simulink model "state_feedback_discrete"  (R2015b)
settings: Solver=VariableStepAuto  StartTime=0.0  StopTime=t  RelTol=1e-3
values from neighbouring files (symbols this model uses):
  A12 = A(1:3,4:6)    [StateSpace.m]
  F = Fe(:,1:size(A,2))    [StateSpace.m]
  FI = Fe(:,size(A,2)+1:size(Fe,2))    [StateSpace.m]
  Jx = 0.0107    [Parameters.m]
  Jy = 0.0107    [Parameters.m]
  Jz = 0.02135    [Parameters.m]
  kd = 9.39741e-7    (= 9.39741e-07)    [Parameters.m]
  kth = 1.32922e-5    (= 1.32922e-05)    [Parameters.m]
  L = 0.225    [Parameters.m]
  Lobs = (-place(A22',A12',[-20 -25 -30]))'    [StateSpace.m]
  pitch_ref = 0.5    [plotSim.m]
  pitch_time = 2    [plotSim.m]
  roll_ref = 0.5    [plotSim.m]
  roll_time = 0.5    [plotSim.m]
  T = 0.035    [plotSim.m]
  w2_bar = sqrt(Fg/kth/4)+1    [Parameters.m]
  w3_bar = sqrt(Fg/kth/4)+1    [Parameters.m]
  w4_bar = sqrt(Fg/kth/4)+1    [Parameters.m]
  yaw_ref = 0.5    [plotSim.m]
  yaw_time = 4    [plotSim.m]
settings Model: Creator=USUARIO  LastModifiedBy=USUARIO

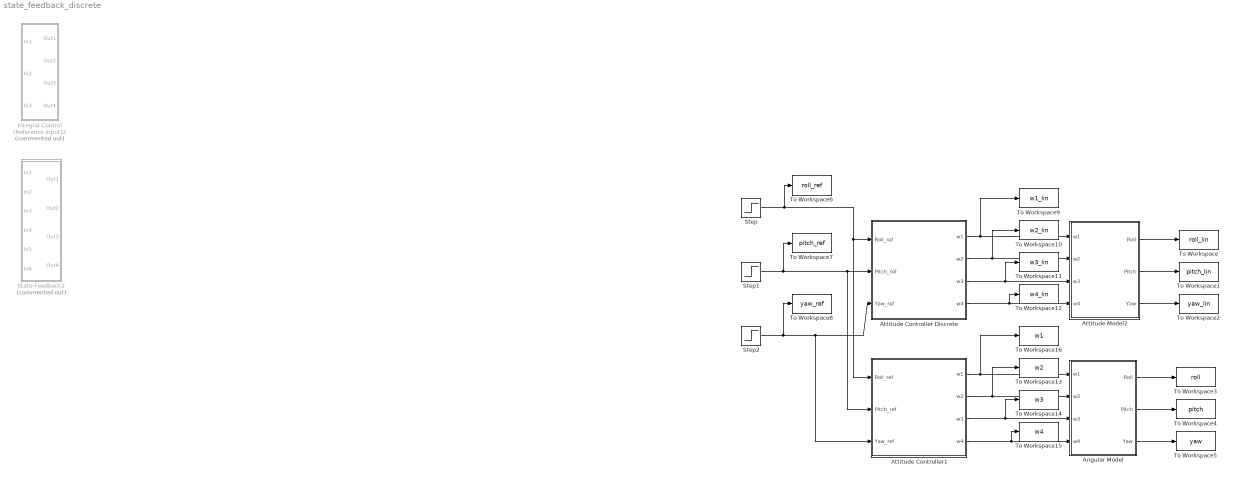
== system state_feedback_discrete ==
  Angular Model : Subsystem
  Attitude Controller Discrete : Subsystem
  Attitude Controller1 : Subsystem
  "Attitude Model2 " : Subsystem
  Integral Control (Reference Input)2 : Subsystem  Commented=on
  State-Feedback2 : Subsystem  Commented=on
  Step : Step  Time=roll_time  After=roll_ref  SampleTime=0
  Step1 : Step  Time=pitch_time  After=pitch_ref  SampleTime=0
  Step2 : Step  Time=yaw_time  After=yaw_ref  SampleTime=0
  To Workspace : ToWorkspace  VariableName=roll_lin  SaveFormat=Timeseries  SampleTime=-1
  To Workspace1 : ToWorkspace  VariableName=pitch_lin  SaveFormat=Timeseries  SampleTime=-1
  To Workspace10 : ToWorkspace  VariableName=w2_lin  SaveFormat=Timeseries  SampleTime=-1
  To Workspace11 : ToWorkspace  VariableName=w3_lin  SaveFormat=Timeseries  SampleTime=-1
  To Workspace12 : ToWorkspace  VariableName=w4_lin  SaveFormat=Timeseries  SampleTime=-1
  To Workspace13 : ToWorkspace  VariableName=w2  SaveFormat=Timeseries  SampleTime=-1
  To Workspace14 : ToWorkspace  VariableName=w3  SaveFormat=Timeseries  SampleTime=-1
  To Workspace15 : ToWorkspace  VariableName=w4  SaveFormat=Timeseries  SampleTime=-1
  To Workspace16 : ToWorkspace  VariableName=w1  SaveFormat=Timeseries  SampleTime=-1
  To Workspace2 : ToWorkspace  VariableName=yaw_lin  SaveFormat=Timeseries  SampleTime=-1
  To Workspace3 : ToWorkspace  VariableName=roll  SaveFormat=Timeseries  SampleTime=-1
  To Workspace4 : ToWorkspace  VariableName=pitch  SaveFormat=Timeseries  SampleTime=-1
  To Workspace5 : ToWorkspace  VariableName=yaw  SaveFormat=Timeseries  SampleTime=-1
  To Workspace6 : ToWorkspace  VariableName=roll_ref  SaveFormat=Timeseries  SampleTime=-1
  To Workspace7 : ToWorkspace  VariableName=pitch_ref  SaveFormat=Timeseries  SampleTime=-1
  To Workspace8 : ToWorkspace  VariableName=yaw_ref  SaveFormat=Timeseries  SampleTime=-1
  To Workspace9 : ToWorkspace  VariableName=w1_lin  SaveFormat=Timeseries  SampleTime=-1
  wires:
  Attitude Controller Discrete/3(w3) -> "Attitude Model2 "/3(w3), To Workspace11/1
  Attitude Controller Discrete/2(w2) -> To Workspace10/1, "Attitude Model2 "/2(w2)
  Attitude Controller Discrete/1(w1) -> To Workspace9/1, "Attitude Model2 "/1(w1)
  Attitude Controller Discrete/4(w4) -> "Attitude Model2 "/4(w4), To Workspace12/1
  "Attitude Model2 "/2(Pitch) -> To Workspace1/1
  "Attitude Model2 "/1(Roll) -> To Workspace/1
  "Attitude Model2 "/3(Yaw) -> To Workspace2/1
  Step/1 -> Attitude Controller1/1(Roll_ref), Attitude Controller Discrete/1(Roll_ref), To Workspace6/1
  Step1/1 -> Attitude Controller1/2(Pitch_ref), Attitude Controller Discrete/2(Pitch_ref), To Workspace7/1
  Step2/1 -> Attitude Controller1/3(Yaw_ref), Attitude Controller Discrete/3(Yaw_ref), To Workspace8/1
  Angular Model/3(Yaw) -> To Workspace5/1
  Angular Model/2(Pitch) -> To Workspace4/1
  Angular Model/1(Roll) -> To Workspace3/1
  Attitude Controller1/3(w3) -> Angular Model/3(w3), To Workspace14/1
  Attitude Controller1/2(w2) -> Angular Model/2(w2), To Workspace13/1
  Attitude Controller1/1(w1) -> To Workspace16/1, Angular Model/1(w1)
  Attitude Controller1/4(w4) -> To Workspace15/1, Angular Model/4(w4)

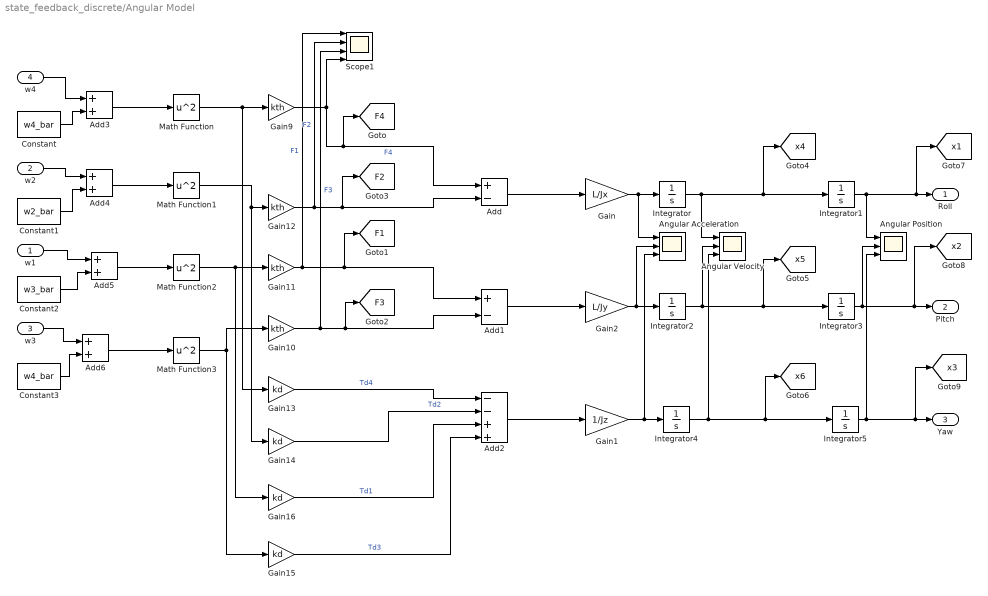
== system state_feedback_discrete/Angular Model ==
  w1 : Inport
  w2 : Inport  Port=2
  w3 : Inport  Port=3
  w4 : Inport  Port=4
  Add : Sum  Inputs=+-
  Add1 : Sum  Inputs=+-
  Add2 : Sum  Inputs=--++
  Add{3..6} (4 alike) : Sum
  Angular Position : Scope  NumInputPorts=3
  Angular Velocity : Scope  NumInputPorts=3
  Angular Acceleration : Scope  NumInputPorts=3
  Constant : Constant  Value=w4_bar
  Constant1 : Constant  Value=w2_bar
  Constant2 : Constant  Value=w3_bar
  Constant3 : Constant  Value=w4_bar
  Gain : Gain  Gain=L/Jx
  Gain1 : Gain  Gain=1/Jz
  Gain{9..12} (4 alike) : Gain  Gain=kth
  Gain{13..16} (4 alike) : Gain  Gain=kd
  Gain2 : Gain  Gain=L/Jy
  Integrator{,1..5} (6 alike) : Integrator
  Math Function{,1..3} (4 alike) : Math  Operator=square  SaturateOnIntegerOverflow=on
  Scope1 : Scope  NumInputPorts=4
  Roll : Outport
  Pitch : Outport  Port=2
  Yaw : Outport  Port=3
  tag scope: F1=global, F2=global, F3=global, F4=global, x1=global, x2=global, x3=global, x4=global, x5=global, x6=global
  wires:
  Gain2/1 -> Angular Acceleration/2, Integrator2/1
  Add2/1 -> Gain1/1
  Gain9/1 -> [F4], Add/1, Scope1/4  "F4"
  Gain14/1 -> Add2/2  "Td2"
  Gain16/1 -> Add2/3  "Td1"
  Gain/1 -> Angular Acceleration/1, Integrator/1
  Integrator/1 -> Angular Velocity/1, Integrator1/1, [x4]
  Integrator1/1 -> [x1], Roll/1, Angular Position/1
  Integrator4/1 -> Angular Velocity/3, [x6], Integrator5/1
  Add/1 -> Gain/1
  Integrator3/1 -> [x2], Pitch/1, Angular Position/2
  Add1/1 -> Gain2/1
  Integrator5/1 -> Angular Position/3, [x3], Yaw/1
  Gain12/1 -> Scope1/2, [F2], Add/2  "F2"
  Gain10/1 -> [F3], Add1/2, Scope1/3  "F3"
  Gain11/1 -> Scope1/1, [F1], Add1/1  "F1"
  Gain13/1 -> Add2/1  "Td4"
  Gain15/1 -> Add2/4  "Td3"
  Integrator2/1 -> Angular Velocity/2, [x5], Integrator3/1
  Gain1/1 -> Angular Acceleration/3, Integrator4/1
  Math Function3/1 -> Gain10/1, Gain15/1
  Math Function2/1 -> Gain16/1, Gain11/1
  Math Function/1 -> Gain13/1, Gain9/1
  Math Function1/1 -> Gain14/1, Gain12/1
  w4/1 -> Add3/1
  Add3/1 -> Math Function/1
  Constant/1 -> Add3/2
  w2/1 -> Add4/1
  Add4/1 -> Math Function1/1
  Constant1/1 -> Add4/2
  w1/1 -> Add5/1
  Add5/1 -> Math Function2/1
  Constant2/1 -> Add5/2
  w3/1 -> Add6/1
  Add6/1 -> Math Function3/1
  Constant3/1 -> Add6/2

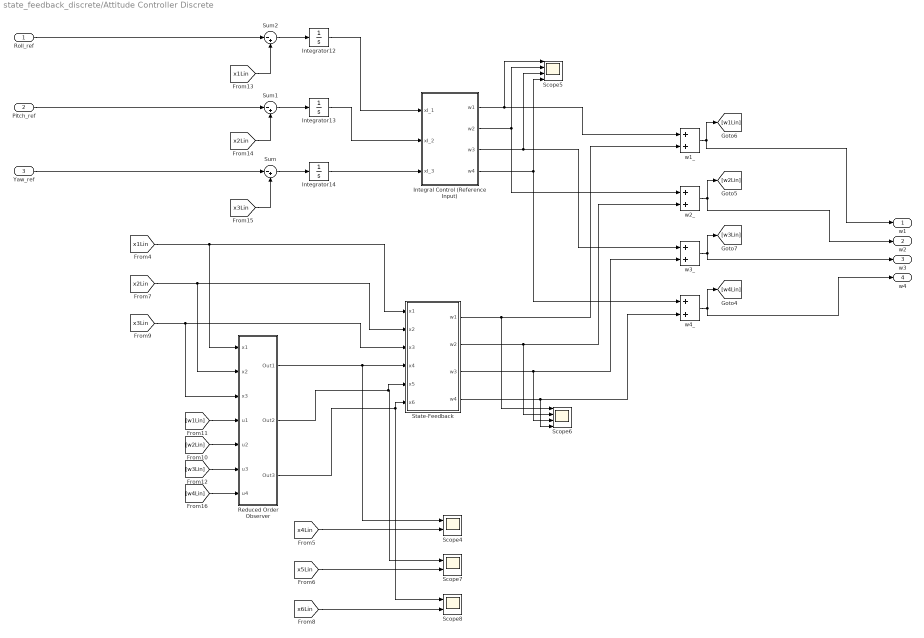
== system state_feedback_discrete/Attitude Controller Discrete ==
  Roll_ref : Inport
  Pitch_ref : Inport  Port=2
  Yaw_ref : Inport  Port=3
  Integral Control (Reference Input) : MATLAB Function  TreatAsAtomicUnit=on
  Integrator12 : Integrator
  Integrator13 : Integrator
  Integrator14 : Integrator
  Reduced Order Observer : Subsystem
  Scope4 : Scope  NumInputPorts=2
  Scope5 : Scope  NumInputPorts=4
  Scope6 : Scope  NumInputPorts=4
  Scope7 : Scope  NumInputPorts=2
  Scope8 : Scope  NumInputPorts=2
  "State-Feedback " : MATLAB Function  TreatAsAtomicUnit=on
  Sum : Sum  Inputs=|-+
  Sum1 : Sum  Inputs=|-+
  Sum2 : Sum  Inputs=|-+
  w1_ : Sum
  w2_ : Sum
  w3_ : Sum
  w4_ : Sum
  w1 : Outport
  w2 : Outport  Port=2
  w3 : Outport  Port=3
  w4 : Outport  Port=4
  wires:
  "State-Feedback "/4(w4) -> w4_/2, Scope6/4
  Roll_ref/1 -> Sum2/1
  [x3Lin] -> Sum/2
  [x1Lin] -> Sum2/2
  Integrator13/1 -> Integral Control (Reference Input)/2(xI_2)
  "State-Feedback "/1(w1) -> w1_/2, Scope6/1
  [w3Lin] -> Reduced Order Observer/6(u3)
  Sum2/1 -> Integrator12/1
  Sum/1 -> Integrator14/1
  [x3Lin] -> "State-Feedback "/3(x3), Reduced Order Observer/3(x3)
  [w2Lin] -> Reduced Order Observer/5(u2)
  Pitch_ref/1 -> Sum1/1
  Integrator14/1 -> Integral Control (Reference Input)/3(xI_3)
  Reduced Order Observer/3(Out3) -> "State-Feedback "/6(x6), Scope8/1
  [x4Lin] -> Scope4/2
  [x6Lin] -> Scope8/2
  "State-Feedback "/2(w2) -> w2_/2, Scope6/2
  Integral Control (Reference Input)/2(w2) -> Scope5/2, w2_/1
  [w4Lin] -> Reduced Order Observer/7(u4)
  Integral Control (Reference Input)/3(w3) -> w3_/1, Scope5/3
  Reduced Order Observer/2(Out2) -> "State-Feedback "/5(x5), Scope7/1
  [x1Lin] -> "State-Feedback "/1(x1), Reduced Order Observer/1(x1)
  [w1Lin] -> Reduced Order Observer/4(u1)
  Integrator12/1 -> Integral Control (Reference Input)/1(xI_1)
  [x2Lin] -> Sum1/2
  Integral Control (Reference Input)/4(w4) -> Scope5/4, w4_/1
  Integral Control (Reference Input)/1(w1) -> w1_/1, Scope5/1
  [x2Lin] -> "State-Feedback "/2(x2), Reduced Order Observer/2(x2)
  Reduced Order Observer/1(Out1) -> "State-Feedback "/4(x4), Scope4/1
  [x5Lin] -> Scope7/2
  Sum1/1 -> Integrator13/1
  Yaw_ref/1 -> Sum/1
  "State-Feedback "/3(w3) -> w3_/2, Scope6/3
  w1_/1 -> w1/1, [w1Lin]
  w4_/1 -> w4/1, [w4Lin]
  w2_/1 -> w2/1, [w2Lin]
  w3_/1 -> w3/1, [w3Lin]

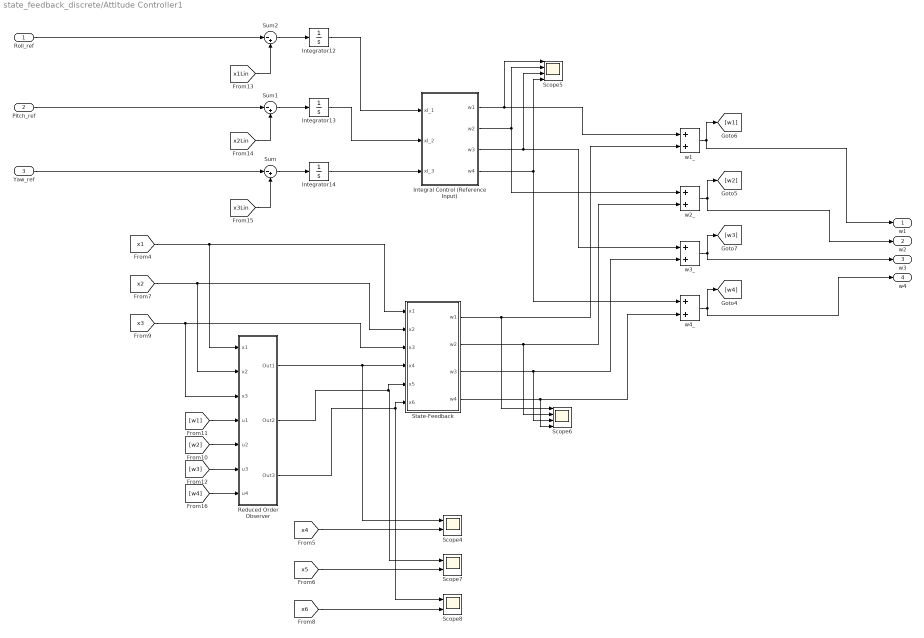
== system state_feedback_discrete/Attitude Controller1 ==
  Roll_ref : Inport
  Pitch_ref : Inport  Port=2
  Yaw_ref : Inport  Port=3
  Integral Control (Reference Input) : MATLAB Function  TreatAsAtomicUnit=on
  Integrator12 : Integrator
  Integrator13 : Integrator
  Integrator14 : Integrator
  Reduced Order Observer : Subsystem
  Scope4 : Scope  NumInputPorts=2
  Scope5 : Scope  NumInputPorts=4
  Scope6 : Scope  NumInputPorts=4
  Scope7 : Scope  NumInputPorts=2
  Scope8 : Scope  NumInputPorts=2
  "State-Feedback " : MATLAB Function  TreatAsAtomicUnit=on
  Sum : Sum  Inputs=|-+
  Sum1 : Sum  Inputs=|-+
  Sum2 : Sum  Inputs=|-+
  w1_ : Sum
  w2_ : Sum
  w3_ : Sum
  w4_ : Sum
  w1 : Outport
  w2 : Outport  Port=2
  w3 : Outport  Port=3
  w4 : Outport  Port=4
  wires:
  w3_/1 -> [w3], w3/1
  w2_/1 -> [w2], w2/1
  w4_/1 -> [w4], w4/1
  w1_/1 -> [w1], w1/1
  "State-Feedback "/3(w3) -> Scope6/3, w3_/2
  Yaw_ref/1 -> Sum/1
  Sum1/1 -> Integrator13/1
  [x5] -> Scope7/2
  Reduced Order Observer/1(Out1) -> Scope4/1, "State-Feedback "/4(x4)
  [x2] -> Reduced Order Observer/2(x2), "State-Feedback "/2(x2)
  Integral Control (Reference Input)/1(w1) -> Scope5/1, w1_/1
  Integral Control (Reference Input)/4(w4) -> w4_/1, Scope5/4
  [x2Lin] -> Sum1/2
  Integrator12/1 -> Integral Control (Reference Input)/1(xI_1)
  [w1] -> Reduced Order Observer/4(u1)
  [x1] -> Reduced Order Observer/1(x1), "State-Feedback "/1(x1)
  Reduced Order Observer/2(Out2) -> Scope7/1, "State-Feedback "/5(x5)
  Integral Control (Reference Input)/3(w3) -> Scope5/3, w3_/1
  [w4] -> Reduced Order Observer/7(u4)
  Integral Control (Reference Input)/2(w2) -> w2_/1, Scope5/2
  "State-Feedback "/2(w2) -> Scope6/2, w2_/2
  [x6] -> Scope8/2
  [x4] -> Scope4/2
  Reduced Order Observer/3(Out3) -> Scope8/1, "State-Feedback "/6(x6)
  Integrator14/1 -> Integral Control (Reference Input)/3(xI_3)
  Pitch_ref/1 -> Sum1/1
  [w2] -> Reduced Order Observer/5(u2)
  [x3] -> Reduced Order Observer/3(x3), "State-Feedback "/3(x3)
  Sum/1 -> Integrator14/1
  Sum2/1 -> Integrator12/1
  [w3] -> Reduced Order Observer/6(u3)
  "State-Feedback "/1(w1) -> Scope6/1, w1_/2
  Integrator13/1 -> Integral Control (Reference Input)/2(xI_2)
  [x1Lin] -> Sum2/2
  [x3Lin] -> Sum/2
  Roll_ref/1 -> Sum2/1
  "State-Feedback "/4(w4) -> Scope6/4, w4_/2

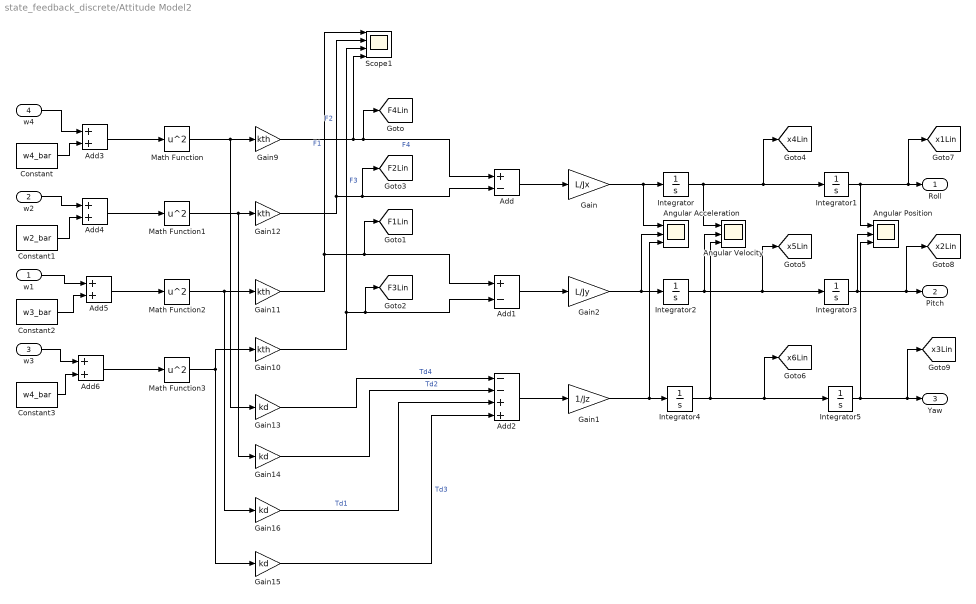
== system state_feedback_discrete/Attitude Model2  ==
  w1 : Inport
  w2 : Inport  Port=2
  w3 : Inport  Port=3
  w4 : Inport  Port=4
  Add : Sum  Inputs=+-
  Add1 : Sum  Inputs=+-
  Add2 : Sum  Inputs=--++
  Add{3..6} (4 alike) : Sum
  Angular Position : Scope  NumInputPorts=3
  Angular Velocity : Scope  NumInputPorts=3
  Angular Acceleration : Scope  NumInputPorts=3
  Constant : Constant  Value=w4_bar
  Constant1 : Constant  Value=w2_bar
  Constant2 : Constant  Value=w3_bar
  Constant3 : Constant  Value=w4_bar
  Gain : Gain  Gain=L/Jx
  Gain1 : Gain  Gain=1/Jz
  Gain{9..12} (4 alike) : Gain  Gain=kth
  Gain{13..16} (4 alike) : Gain  Gain=kd
  Gain2 : Gain  Gain=L/Jy
  Integrator{,1..5} (6 alike) : Integrator
  Math Function{,1..3} (4 alike) : Math  Operator=square  SaturateOnIntegerOverflow=on
  Scope1 : Scope  NumInputPorts=4
  Roll : Outport
  Pitch : Outport  Port=2
  Yaw : Outport  Port=3
  tag scope: F1Lin=global, F2Lin=global, F3Lin=global, F4Lin=global, x1Lin=global, x2Lin=global, x3Lin=global, x4Lin=global, x5Lin=global, x6Lin=global
  wires:
  Gain1/1 -> Integrator4/1, Angular Acceleration/3
  Integrator2/1 -> Integrator3/1, [x5Lin], Angular Velocity/2
  Gain15/1 -> Add2/4  "Td3"
  Gain13/1 -> Add2/1  "Td4"
  Gain11/1 -> Add1/1, [F1Lin], Scope1/1  "F1"
  Gain10/1 -> Scope1/3, Add1/2, [F3Lin]  "F3"
  Gain12/1 -> Scope1/2, Add/2, [F2Lin]  "F2"
  Integrator5/1 -> Yaw/1, [x3Lin], Angular Position/3
  Add1/1 -> Gain2/1
  Integrator3/1 -> Angular Position/2, Pitch/1, [x2Lin]
  Add/1 -> Gain/1
  Integrator4/1 -> Integrator5/1, [x6Lin], Angular Velocity/3
  Integrator1/1 -> Angular Position/1, Roll/1, [x1Lin]
  Integrator/1 -> [x4Lin], Integrator1/1, Angular Velocity/1
  Gain/1 -> Integrator/1, Angular Acceleration/1
  Gain16/1 -> Add2/3  "Td1"
  Gain14/1 -> Add2/2  "Td2"
  Gain9/1 -> Scope1/4, Add/1, [F4Lin]  "F4"
  Add2/1 -> Gain1/1
  Gain2/1 -> Integrator2/1, Angular Acceleration/2
  Math Function3/1 -> Gain10/1, Gain15/1
  Math Function2/1 -> Gain16/1, Gain11/1
  Math Function/1 -> Gain13/1, Gain9/1
  Math Function1/1 -> Gain14/1, Gain12/1
  w4/1 -> Add3/1
  Add3/1 -> Math Function/1
  Constant/1 -> Add3/2
  w2/1 -> Add4/1
  Add4/1 -> Math Function1/1
  Constant1/1 -> Add4/2
  w1/1 -> Add5/1
  Add5/1 -> Math Function2/1
  Constant2/1 -> Add5/2
  w3/1 -> Add6/1
  Add6/1 -> Math Function3/1
  Constant3/1 -> Add6/2

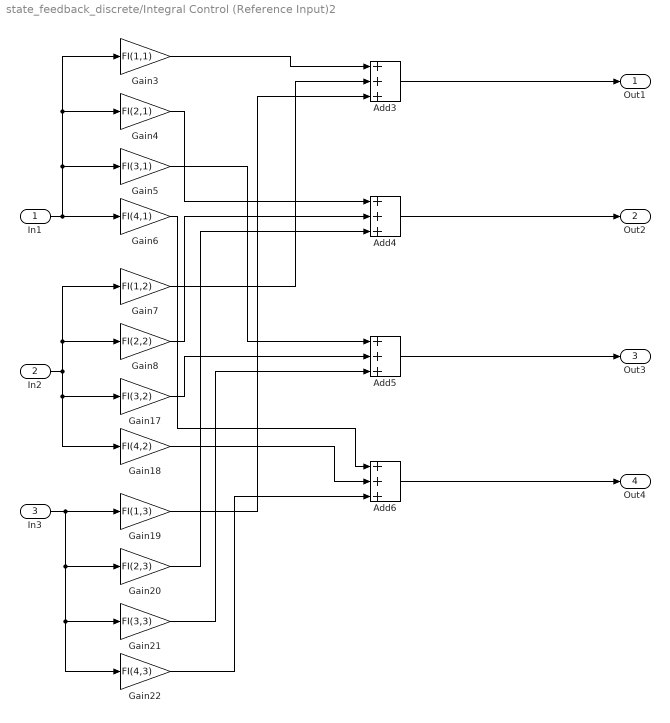
== system state_feedback_discrete/Integral Control (Reference Input)2 ==
  In1 : Inport
  In2 : Inport  Port=2
  In3 : Inport  Port=3
  Add{3..6} (4 alike) : Sum  Inputs=+++
  Gain17 : Gain  Gain=FI(3,2)
  Gain18 : Gain  Gain=FI(4,2)
  Gain19 : Gain  Gain=FI(1,3)
  Gain20 : Gain  Gain=FI(2,3)
  Gain21 : Gain  Gain=FI(3,3)
  Gain22 : Gain  Gain=FI(4,3)
  Gain3 : Gain  Gain=FI(1,1)
  Gain4 : Gain  Gain=FI(2,1)
  Gain5 : Gain  Gain=FI(3,1)
  Gain6 : Gain  Gain=FI(4,1)
  Gain7 : Gain  Gain=FI(1,2)
  Gain8 : Gain  Gain=FI(2,2)
  Out1 : Outport
  Out2 : Outport  Port=2
  Out3 : Outport  Port=3
  Out4 : Outport  Port=4
  wires:
  Gain21/1 -> Add5/3
  Gain17/1 -> Add5/2
  Gain5/1 -> Add5/1
  Gain6/1 -> Add6/1
  Gain22/1 -> Add6/3
  Gain18/1 -> Add6/2
  In2/1 -> Gain7/1, Gain8/1, Gain17/1, Gain18/1
  Add5/1 -> Out3/1
  Add6/1 -> Out4/1
  In3/1 -> Gain19/1, Gain20/1, Gain22/1, Gain21/1
  Add3/1 -> Out1/1
  Add4/1 -> Out2/1
  Gain20/1 -> Add4/3
  Gain3/1 -> Add3/1
  Gain19/1 -> Add3/3
  Gain7/1 -> Add3/2
  Gain8/1 -> Add4/2
  Gain4/1 -> Add4/1
  In1/1 -> Gain3/1, Gain4/1, Gain5/1, Gain6/1

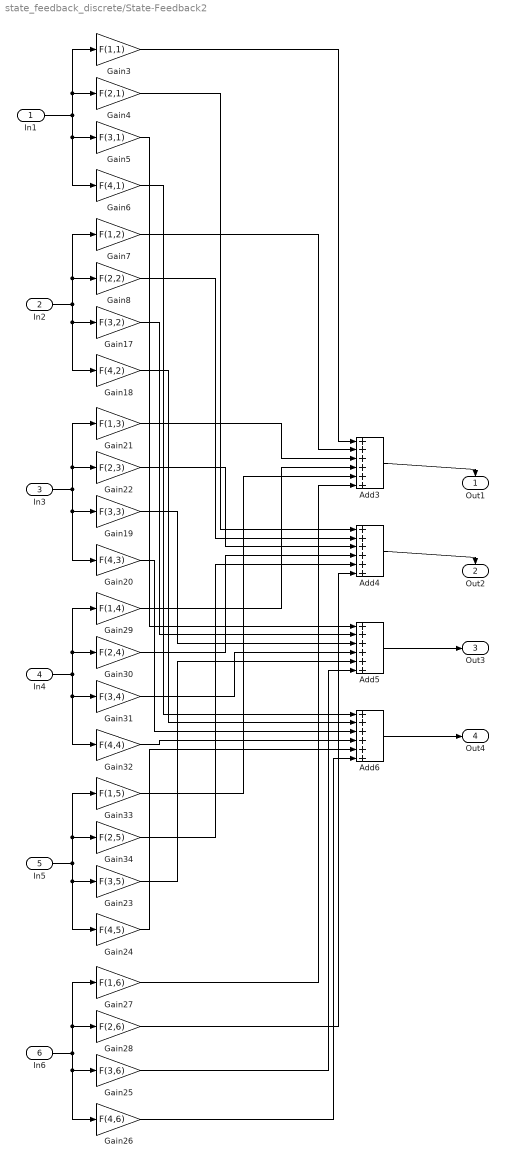
== system state_feedback_discrete/State-Feedback2 ==
  In1 : Inport
  In2 : Inport  Port=2
  In3 : Inport  Port=3
  In4 : Inport  Port=4
  In5 : Inport  Port=5
  In6 : Inport  Port=6
  Add{3..6} (4 alike) : Sum  Inputs=++++++
  Gain17 : Gain  Gain=F(3,2)
  Gain18 : Gain  Gain=F(4,2)
  Gain19 : Gain  Gain=F(3,3)
  Gain20 : Gain  Gain=F(4,3)
  Gain21 : Gain  Gain=F(1,3)
  Gain22 : Gain  Gain=F(2,3)
  Gain23 : Gain  Gain=F(3,5)
  Gain24 : Gain  Gain=F(4,5)
  Gain25 : Gain  Gain=F(3,6)
  Gain26 : Gain  Gain=F(4,6)
  Gain27 : Gain  Gain=F(1,6)
  Gain28 : Gain  Gain=F(2,6)
  Gain29 : Gain  Gain=F(1,4)
  Gain3 : Gain  Gain=F(1,1)
  Gain30 : Gain  Gain=F(2,4)
  Gain31 : Gain  Gain=F(3,4)
  Gain32 : Gain  Gain=F(4,4)
  Gain33 : Gain  Gain=F(1,5)
  Gain34 : Gain  Gain=F(2,5)
  Gain4 : Gain  Gain=F(2,1)
  Gain5 : Gain  Gain=F(3,1)
  Gain6 : Gain  Gain=F(4,1)
  Gain7 : Gain  Gain=F(1,2)
  Gain8 : Gain  Gain=F(2,2)
  Out1 : Outport
  Out2 : Outport  Port=2
  Out3 : Outport  Port=3
  Out4 : Outport  Port=4
  wires:
  In2/1 -> Gain8/1, Gain7/1, Gain18/1, Gain17/1
  In1/1 -> Gain6/1, Gain5/1, Gain4/1, Gain3/1
  In3/1 -> Gain22/1, Gain21/1, Gain20/1, Gain19/1
  In5/1 -> Gain34/1, Gain33/1, Gain24/1, Gain23/1
  In4/1 -> Gain32/1, Gain31/1, Gain30/1, Gain29/1
  In6/1 -> Gain28/1, Gain27/1, Gain26/1, Gain25/1
  Add3/1 -> Out1/1
  Add4/1 -> Out2/1
  Add5/1 -> Out3/1
  Add6/1 -> Out4/1
  Gain4/1 -> Add4/1
  Gain22/1 -> Add4/3
  Gain8/1 -> Add4/2
  Gain34/1 -> Add4/5
  Gain30/1 -> Add4/4
  Gain28/1 -> Add4/6
  Gain24/1 -> Add6/5
  Gain20/1 -> Add6/3
  Gain6/1 -> Add6/1
  Gain18/1 -> Add6/2
  Gain26/1 -> Add6/6
  Gain32/1 -> Add6/4
  Gain7/1 -> Add3/2
  Gain21/1 -> Add3/3
  Gain29/1 -> Add3/4
  Gain27/1 -> Add3/6
  Gain3/1 -> Add3/1
  Gain33/1 -> Add3/5
  Gain23/1 -> Add5/5
  Gain17/1 -> Add5/2
  Gain19/1 -> Add5/3
  Gain5/1 -> Add5/1
  Gain31/1 -> Add5/4
  Gain25/1 -> Add5/6

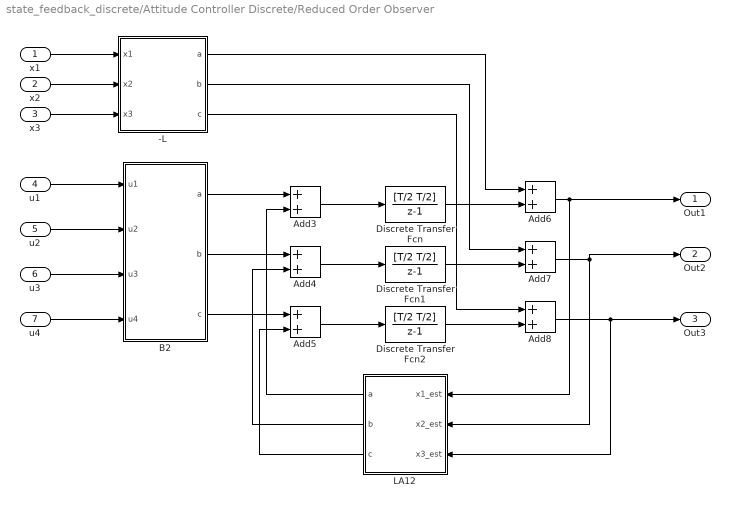
== system state_feedback_discrete/Attitude Controller Discrete/Reduced Order Observer ==
  x1 : Inport
  x2 : Inport  Port=2
  x3 : Inport  Port=3
  u1 : Inport  Port=4
  u2 : Inport  Port=5
  u3 : Inport  Port=6
  u4 : Inport  Port=7
  "-L " : MATLAB Function  TreatAsAtomicUnit=on
  Add{3..8} (6 alike) : Sum  Inputs=2
  B2 : MATLAB Function  TreatAsAtomicUnit=on
  Discrete Transfer Fcn : DiscreteTransferFcn  Numerator=[T/2 T/2]  Denominator=[1 -1]  SampleTime=T
  Discrete Transfer Fcn1 : DiscreteTransferFcn  Numerator=[T/2 T/2]  Denominator=[1 -1]  SampleTime=T
  Discrete Transfer Fcn2 : DiscreteTransferFcn  Numerator=[T/2 T/2]  Denominator=[1 -1]  SampleTime=T
  LA12 : MATLAB Function  TreatAsAtomicUnit=on
  Out1 : Outport
  Out2 : Outport  Port=2
  Out3 : Outport  Port=3
  wires:
  Add4/1 -> Discrete Transfer Fcn1/1
  Add3/1 -> Discrete Transfer Fcn/1
  Add5/1 -> Discrete Transfer Fcn2/1
  u4/1 -> B2/4(u4)
  u2/1 -> B2/2(u2)
  B2/1(a) -> Add3/1
  B2/2(b) -> Add4/1
  B2/3(c) -> Add5/1
  LA12/1(a) -> Add3/2
  LA12/2(b) -> Add4/2
  LA12/3(c) -> Add5/2
  Add6/1 -> LA12/1(x1_est), Out1/1
  Add7/1 -> LA12/2(x2_est), Out2/1
  Add8/1 -> LA12/3(x3_est), Out3/1
  "-L "/3(c) -> Add8/1
  "-L "/1(a) -> Add6/1
  "-L "/2(b) -> Add7/1
  x2/1 -> "-L "/2(x2)
  x3/1 -> "-L "/3(x3)
  x1/1 -> "-L "/1(x1)
  u1/1 -> B2/1(u1)
  u3/1 -> B2/3(u3)
  Discrete Transfer Fcn/1 -> Add6/2
  Discrete Transfer Fcn1/1 -> Add7/2
  Discrete Transfer Fcn2/1 -> Add8/2

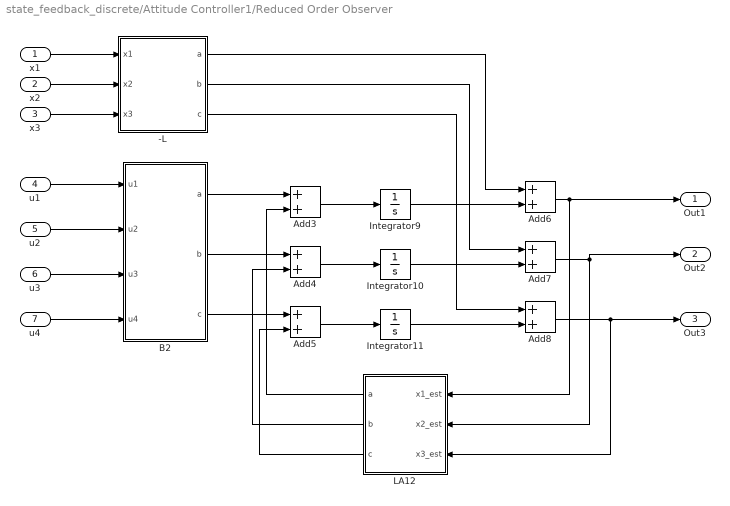
== system state_feedback_discrete/Attitude Controller1/Reduced Order Observer ==
  x1 : Inport
  x2 : Inport  Port=2
  x3 : Inport  Port=3
  u1 : Inport  Port=4
  u2 : Inport  Port=5
  u3 : Inport  Port=6
  u4 : Inport  Port=7
  "-L " : MATLAB Function  TreatAsAtomicUnit=on
  Add{3..8} (6 alike) : Sum  Inputs=2
  B2 : MATLAB Function  TreatAsAtomicUnit=on
  Integrator10 : Integrator
  Integrator11 : Integrator
  Integrator9 : Integrator
  LA12 : MATLAB Function  TreatAsAtomicUnit=on
  Out1 : Outport
  Out2 : Outport  Port=2
  Out3 : Outport  Port=3
  wires:
  u3/1 -> B2/3(u3)
  u1/1 -> B2/1(u1)
  Integrator10/1 -> Add7/2
  Integrator11/1 -> Add8/2
  Integrator9/1 -> Add6/2
  x1/1 -> "-L "/1(x1)
  x3/1 -> "-L "/3(x3)
  x2/1 -> "-L "/2(x2)
  "-L "/2(b) -> Add7/1
  "-L "/1(a) -> Add6/1
  "-L "/3(c) -> Add8/1
  Add8/1 -> Out3/1, LA12/3(x3_est)
  Add7/1 -> Out2/1, LA12/2(x2_est)
  Add6/1 -> Out1/1, LA12/1(x1_est)
  LA12/3(c) -> Add5/2
  LA12/2(b) -> Add4/2
  LA12/1(a) -> Add3/2
  B2/3(c) -> Add5/1
  B2/2(b) -> Add4/1
  B2/1(a) -> Add3/1
  u2/1 -> B2/2(u2)
  u4/1 -> B2/4(u4)
  Add5/1 -> Integrator11/1
  Add3/1 -> Integrator9/1
  Add4/1 -> Integrator10/1

== matlab function state_feedback_discrete/Attitude Controller1/Integral Control (Reference Input) ==
  data: xI_1 input; w1 output; w2 output; w3 output; w4 output; xI_2 input; xI_3 input; FI parameter
function [w1,w2,w3,w4] = FI_matrix(xI_1, xI_2, xI_3,FI)
xI=[xI_1;
    xI_2;
    xI_3];

w=FI*xI;

w1=w(1);
w2=w(2);
w3=w(3);
w4=w(4);

== matlab function state_feedback_discrete/Attitude Controller1/Reduced Order Observer/-L  ==
  data: x1 input; a output; b output; c output; x2 input; x3 input; Lobs parameter
function [a,b,c] = minusL_matrix(x1, x2, x3, Lobs)
x=[x1;
    x2;
    x3];

abc=-Lobs*x;

a=abc(1);
b=abc(2);
c=abc(3);

== matlab function state_feedback_discrete/Attitude Controller1/Reduced Order Observer/B2 ==
  data: u1 input; a output; b output; c output; u2 input; u3 input; u4 input; B2 parameter
function [a, b, c] = B2_matrix(u1, u2, u3, u4, B2)
u=[u1;
    u2;
    u3;
    u4];

abc=B2*u;

a=abc(1);
b=abc(2);
c=abc(3);

== matlab function state_feedback_discrete/Attitude Controller1/Reduced Order Observer/LA12 ==
  data: x1_est input; x2_est input; x3_est input; a output; b output; c output; Lobs parameter; A12 parameter
function [a,b,c] = LA12_matrix(x1_est, x2_est, x3_est, Lobs, A12)
x=[x1_est;
    x2_est;
    x3_est];

abc=Lobs*A12*x;

a=abc(1);
b=abc(2);
c=abc(3);

== matlab function state_feedback_discrete/Attitude Controller1/State-Feedback  ==
  data: x1 input; w1 output; w2 output; w3 output; w4 output; x2 input; x3 input; x4 input; x5 input; x6 input; F parameter
function [w1,w2,w3,w4] = F_matrix(x1, x2, x3, x4, x5, x6, F)
x=[x1;
    x2;
    x3;
    x4;
    x5;
    x6];

w=F*x;

w1=w(1);
w2=w(2);
w3=w(3);
w4=w(4);

== matlab function state_feedback_discrete/Attitude Controller Discrete/Integral Control (Reference Input) ==
  data: xI_1 input; w1 output; w2 output; w3 output; w4 output; xI_2 input; xI_3 input; FI parameter
function [w1,w2,w3,w4] = FI_matrix(xI_1, xI_2, xI_3,FI)
xI=[xI_1;
    xI_2;
    xI_3];

w=FI*xI;

w1=w(1);
w2=w(2);
w3=w(3);
w4=w(4);

== matlab function state_feedback_discrete/Attitude Controller Discrete/Reduced Order Observer/-L  ==
  data: x1 input; a output; b output; c output; x2 input; x3 input; Lobs parameter
function [a,b,c] = minusL_matrix(x1, x2, x3, Lobs)
x=[x1;
    x2;
    x3];

abc=-Lobs*x;

a=abc(1);
b=abc(2);
c=abc(3);

== matlab function state_feedback_discrete/Attitude Controller Discrete/Reduced Order Observer/B2 ==
  data: u1 input; a output; b output; c output; u2 input; u3 input; u4 input; B2 parameter
function [a, b, c] = B2_matrix(u1, u2, u3, u4, B2)
u=[u1;
    u2;
    u3;
    u4];

abc=B2*u;

a=abc(1);
b=abc(2);
c=abc(3);

== matlab function state_feedback_discrete/Attitude Controller Discrete/Reduced Order Observer/LA12 ==
  data: x1_est input; x2_est input; x3_est input; a output; b output; c output; Lobs parameter; A12 parameter
function [a,b,c] = LA12_matrix(x1_est, x2_est, x3_est, Lobs, A12)
x=[x1_est;
    x2_est;
    x3_est];

abc=Lobs*A12*x;

a=abc(1);
b=abc(2);
c=abc(3);

== matlab function state_feedback_discrete/Attitude Controller Discrete/State-Feedback  ==
  data: x1 input; w1 output; w2 output; w3 output; w4 output; x2 input; x3 input; x4 input; x5 input; x6 input; F parameter
function [w1,w2,w3,w4] = F_matrix(x1, x2, x3, x4, x5, x6, F)
x=[x1;
    x2;
    x3;
    x4;
    x5;
    x6];

w=F*x;

w1=w(1);
w2=w(2);
w3=w(3);
w4=w(4);
